simulink model "LQG_r"  (R2023b)
settings: Solver=VariableStepAuto  StartTime=0.0  StopTime=200  RelTol=1e-3
undefined symbols (not defined in the file): A, A_kf, B_kf, B_total, C_kf, C_ss, CI, D_kf, DI, DiscIntNeverNeededParam, Discrete, dVdt, K, Kint, Rn_ext, sigma, step_temp, steptime, Time, Ts, Tsp, Ufeedforward, Vb0, Vmax, Vmin, wd
libraries: simulink x3, ctrlSharedLib x1
settings Model: Creator=Maialen  LastModifiedBy=Maialen

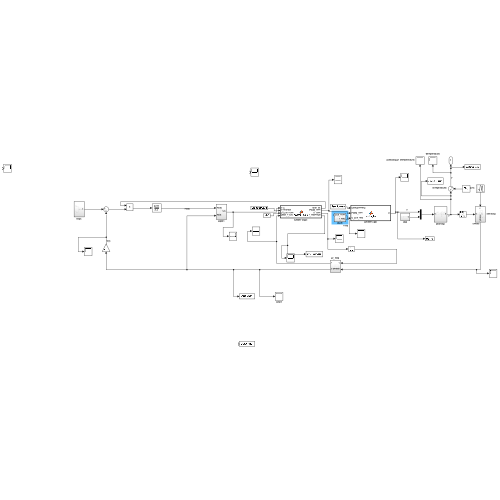
[thumbnail: Simulink's stored preview of the top-level diagram]
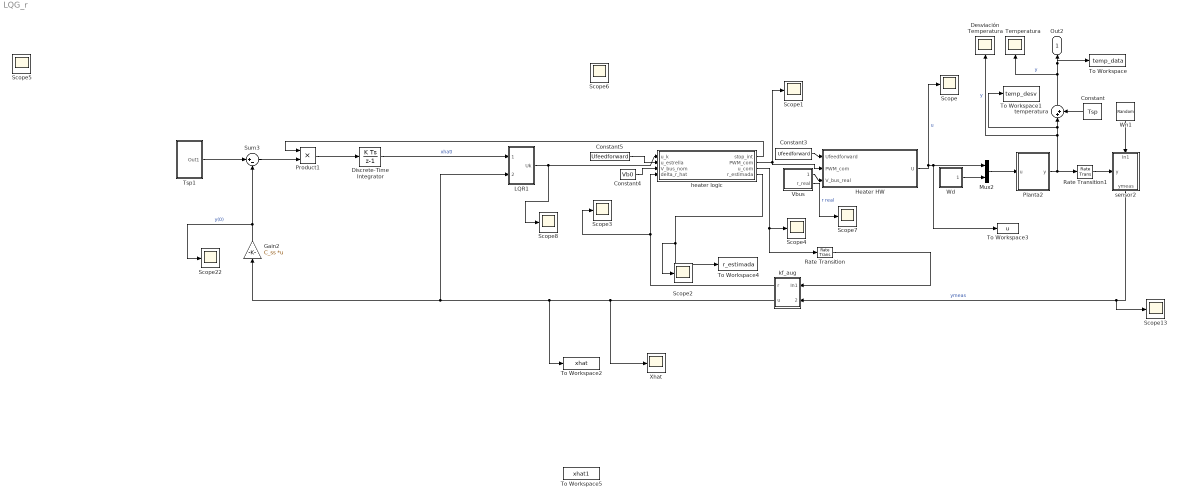
== system LQG_r ==
  Constant : Constant  Value=Tsp  SampleTime=0
  Constant3 : Constant  Value=Ufeedforward  SampleTime=0
  Constant4 : Constant  Value=Vb0  SampleTime=0
  Constant5 : Constant  Value=Ufeedforward  SampleTime=0
  Desviación Temperatura : Scope
  Discrete-Time Integrator : DiscreteIntegrator  SampleTime=Ts  ICPrevOutput=DiscIntNeverNeededParam  ICPrevScaledInput=DiscIntNeverNeededParam
  Gain2 : Gain  Gain=C_ss  Multiplication=Matrix(K*u)
  Heater HW : MATLAB Function  TreatAsAtomicUnit=on
  LQR1 : Subsystem
  Mux2 : Mux  Inputs=2
  Planta2 : Subsystem
  Product1 : Product
  Rate Transition : RateTransition  OutPortSampleTime=Ts
  Rate Transition1 : RateTransition  OutPortSampleTime=Ts
  Scope{,1..8,13,22} (11 alike) : Scope
  Sum3 : Sum  Inputs=|+-
  Temperatura : Scope
  To Workspace : ToWorkspace  VariableName=temp_data  SaveFormat=Timeseries  SampleTime=-1
  To Workspace1 : ToWorkspace  VariableName=temp_desv  SaveFormat=Timeseries  SampleTime=-1
  To Workspace2 : ToWorkspace  VariableName=xhat  SaveFormat=Timeseries  SampleTime=-1
  To Workspace3 : ToWorkspace  VariableName=u  SaveFormat=Timeseries  SampleTime=Ts
  To Workspace4 : ToWorkspace  VariableName=r_estimada  SaveFormat=Timeseries  SampleTime=-1
  To Workspace5 : ToWorkspace  VariableName=xhat1  SaveFormat=Timeseries  SampleTime=-1
  Tsp1 : Subsystem
  Vbus : Subsystem
  Wd : Subsystem
  Wn1 : RandomNumber  Variance=sigma^2  SampleTime=Ts
  Xhat : Scope
  heater logic : MATLAB Function  TreatAsAtomicUnit=on
  kf_aug : Subsystem
  sensor2 : Subsystem
      settings: PortSchema="{\"entries\":[{\"content\":{\"sides\":[{\"content\":{\"connectorIds\":[\"In1\"]},\"type\":\"ConnectorPlacement.EquallySpacedRectSide\",\"uuid\":\"87c57665-5a3a-4a29-be31-fc3b8356ea98\"},{\"content\":{\"connectorIds\":[\"Out1\"],\"side\":\"RIGHT\"},\"type\":\"ConnectorPlacement.EquallySpacedRectSide\",\"uuid\":\"3fe956b0-7f9e-4b46-bcb6-e49be4c7e683\"},{\"content\":{\"connectorIds\":[\"In2\"],\"side\":\"TOP\"},\"type\":\"ConnectorPlacement.EquallySpacedRectSide\",\"uuid\":\"3d207620-bc84-4c0d-9751-3dea453ac424\"}]},\"type\":\"ConnectorPlacement.EquallySpacedConnector\",\"uuid\":\"7e1a59fd-e04d-40d6-8549-9ebaaabea5d7\"}],\"packageUris\":[\"http://schema.mathworks.com/mf0/Connector/R2020b\"],\"version\":\"1.0\"}"
  temperatura : Sum  Inputs=|++
  Out2 : Outport
  wires:
  Vbus/2(r_real) -> Scope7/1  "r real"
  temperatura/1 -> To Workspace/1, Out2/1, Temperatura/1  "y"
  heater logic/3(u_com) -> Scope4/1, Rate Transition/1
  Vbus/1(V_bus_nom) -> Heater HW/3(V_bus_real)
  Heater HW/1(U) -> To Workspace3/1, Mux2/1, Scope/1  "u"
  Rate Transition1/1 -> sensor2/2(y)
  heater logic/4(r_estimada) -> To Workspace4/1, Scope2/1
  Rate Transition/1 -> kf_aug/1(In1)
  Constant3/1 -> Heater HW/1(Ufeedforward)
  Wd/1(Out1) -> Mux2/2
  Mux2/1 -> Planta2/1(u)
  Constant4/1 -> heater logic/3(V_bus_nom)
  Constant/1 -> temperatura/2
  Planta2/1(y) -> Desviación Temperatura/1, To Workspace1/1, temperatura/1, Rate Transition1/1  "y"
  kf_aug/2(u) -> To Workspace2/1, LQR1/2(xhat), Gain2/1, Xhat/1
  heater logic/2(PWM_com) -> Scope1/1, Heater HW/2(PWM_com)
  Constant5/1 -> heater logic/2(u_estrella)
  kf_aug/1(r) -> Scope3/1, heater logic/4(delta_r_hat)
  Wn1/1 -> sensor2/1(In1)
  sensor2/1(ymeas) -> kf_aug/2(ymeas), Scope13/1  "ymeas"
  LQR1/1(Uk) -> Scope8/1, heater logic/1(u_k)
  Discrete-Time Integrator/1 -> LQR1/1(xhatI)  "xhatI"
  Tsp1/1(Out1) -> Sum3/1
  Product1/1 -> Discrete-Time Integrator/1
  Sum3/1 -> Product1/2
  Gain2/1 -> Sum3/2, Scope22/1  "y(0)"
  heater logic/1(stop_int) -> Product1/1

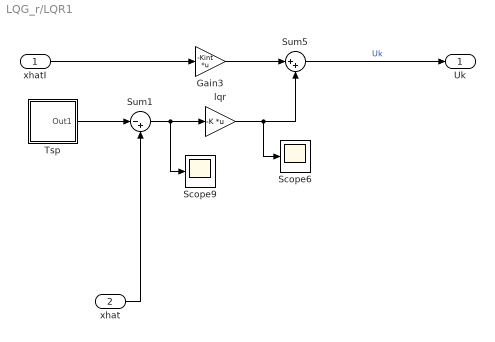
== system LQG_r/LQR1 ==
  xhatI : Inport
  xhat : Inport  Port=2
  Gain3 : Gain  Gain=-Kint  Multiplication=Matrix(K*u)
  Scope6 : Scope
  Scope9 : Scope
  Sum1 : Sum  Inputs=|-+
  Sum5 : Sum  Inputs=|++
  Tsp : Subsystem
  lqr : Gain  Gain=-K  Multiplication=Matrix(K*u)
  Uk : Outport
  wires:
  xhatI/1 -> Gain3/1
  lqr/1 -> Scope6/1, Sum5/2
  Gain3/1 -> Sum5/1
  Sum1/1 -> Scope9/1, lqr/1
  xhat/1 -> Sum1/2
  Tsp/1(Out1) -> Sum1/1
  Sum5/1 -> Uk/1  "Uk"

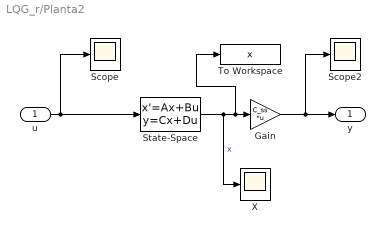
== system LQG_r/Planta2 ==
  u : Inport
  Gain : Gain  Gain=C_ss  Multiplication=Matrix(K*u)
  Scope : Scope
  Scope2 : Scope
  State-Space : StateSpace  A=A  B=B_total  C=CI  D=DI  InitialCondition=0
  To Workspace : ToWorkspace  VariableName=x  SaveFormat=Timeseries  SampleTime=-1
  X : Scope
  y : Outport
  wires:
  Gain/1 -> Scope2/1, y/1
  State-Space/1 -> X/1, To Workspace/1, Gain/1  "x"
  u/1 -> State-Space/1, Scope/1

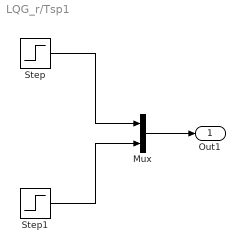
== system LQG_r/Tsp1 ==
  Mux : Mux  Inputs=2
  Step : Step  Time=steptime  After=step_temp  SampleTime=0
  Step1 : Step  Time=steptime  After=step_temp  SampleTime=0
  Out1 : Outport
  wires:
  Mux/1 -> Out1/1
  Step/1 -> Mux/1
  Step1/1 -> Mux/2

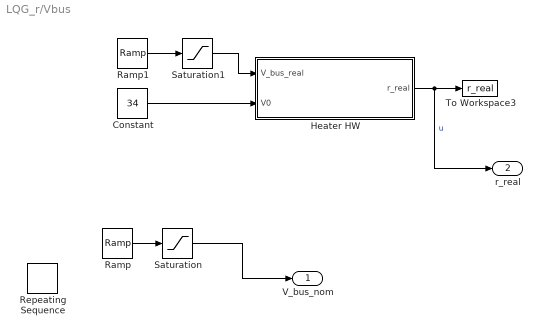
== system LQG_r/Vbus ==
  Constant : Constant  Value=34  SampleTime=0
  Heater HW : MATLAB Function  TreatAsAtomicUnit=on
  Ramp : simulink/Sources/Ramp  slope=dVdt  start=steptime  InitialOutput=Vb0
  Ramp1 : simulink/Sources/Ramp  slope=dVdt  start=steptime  InitialOutput=34
  Repeating Sequence : simulink/Sources/Repeating Sequence  rep_seq_t=[0, 20, 110, 310, 400, 600, 690, 890, 980]  rep_seq_y=[34, 34, 28, 28, 34, 34, 28, 28, 34]
  Saturation : Saturate  UpperLimit=Vmax  LowerLimit=Vmin
  Saturation1 : Saturate  UpperLimit=Vmax  LowerLimit=Vmin
  To Workspace3 : ToWorkspace  VariableName=r_real  SaveFormat=Timeseries  SampleTime=-1
  V_bus_nom : Outport
  r_real : Outport  Port=2
  wires:
  Constant/1 -> Heater HW/2(V0)
  Heater HW/1(r_real) -> r_real/1, To Workspace3/1  "u"
  Ramp/1 -> Saturation/1
  Saturation1/1 -> Heater HW/1(V_bus_real)
  Ramp1/1 -> Saturation1/1
  Saturation/1 -> V_bus_nom/1

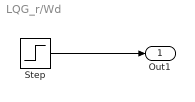
== system LQG_r/Wd ==
  Step : Step  Time=steptime  After=wd  SampleTime=0
  Out1 : Outport
  wires:
  Step/1 -> Out1/1

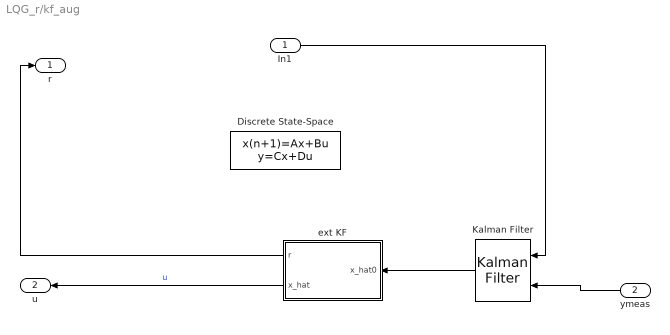
== system LQG_r/kf_aug ==
  In1 : Inport
  ymeas : Inport  Port=2
  Discrete State-Space : DiscreteStateSpace  A=A_kf  B=B_kf  C=C_kf  D=D_kf  SampleTime=Ts
  Kalman Filter : ctrlSharedLib/Kalman Filter  TimeDomain=Discrete-Time  UseCurrentEstimator=on  ModelSource=LTI State-Space Variable  ModelSourceVariable=syskf_ext  A=0.95  B=1  C=1  D=0  NumberOfStates=1  NumberOfInputs=1  NumberOfOutputs=1  InitialEstimateSource=Dialog  X0=0  P0=10  UseK=off  UseGH=off  NumberOfProcessNoiseInputs=1  G=1  TimeInvariantG=on  H=0  TimeInvariantH=on  Q=Qn_ext  TimeInvariantQ=on  R=Rn_ext  TimeInvariantR=on  N=0  TimeInvariantN=on  AddInputPort=on  AddEnablePort=off  OutputEstimatedY=off  OutputP=off  Ts=-1
  ext KF : MATLAB Function  TreatAsAtomicUnit=on
  r : Outport
  u : Outport  Port=2
  wires:
  ext KF/2(x_hat) -> u/1  "u"
  ext KF/1(r) -> r/1
  ymeas/1 -> Kalman Filter/2
  In1/1 -> Kalman Filter/1
  Kalman Filter/1 -> ext KF/1(x_hat0)

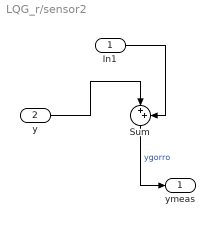
== system LQG_r/sensor2 ==
  In1 : Inport
  y : Inport  Port=2
  Sum : Sum  Inputs=|++
  ymeas : Outport
  wires:
  In1/1 -> Sum/2
  y/1 -> Sum/1
  Sum/1 -> ymeas/1  "ygorro"

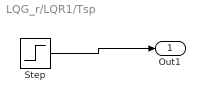
== system LQG_r/LQR1/Tsp ==
  Step : Step  Time=steptime  After=step_temp  SampleTime=0
  Out1 : Outport
  wires:
  Step/1 -> Out1/1

== matlab function LQG_r/Heater HW ==
  data: Ufeedforward input; PWM_com input; U output; V_bus_real input
function U = heater_hw(Ufeedforward, PWM_com, V_bus_real)
    R_real = [156.8; 156.8];
    
    % Potencia real entregada a la planta
    P_max_real = (V_bus_real^2) ./ R_real;
    U= PWM_com .* P_max_real - Ufeedforward;
end

== matlab function LQG_r/kf_aug/ext KF ==
  data: r output; x_hat0 input; x_hat output
function [r, x_hat] = ext(x_hat0)
   % x_hat es la salida del filtro (39x1)
x_hat = x_hat0(1:38); 
r = (x_hat0(39) ) ;

end

== matlab function LQG_r/Vbus/Heater HW ==
  data: V_bus_real input; V0 input; r_real output
function r_real = eficiencia_real(V_bus_real, V0)
    R_real = [156.8; 156.8];
    r_real = (V_bus_real/V0)^2;
end

== matlab function LQG_r/heater logic ==
  data: stop_int output; u_k input; u_estrella input; PWM_com output; V_bus_nom input; delta_r_hat input; u_com output; r_estimada output
function [stop_int, PWM_com, u_com, r_estimada] = heater_logic(u_k, u_estrella, V_bus_nom, delta_r_hat)
% u_k        : salida del controlador LQR (desviación de control)
% u_estrella : feedforward nominal (Ufeedforward)
% V_bus_nom  : voltaje nominal del bus (34V)
% delta_r_hat: estimación de Δr = r-1 del Kalman aumentado

    R0 = [156.8; 156.8];
    P_max_nom = (V_bus_nom^2) ./ R0;   % potencia máxima en nominal

   

    % Compensación feedforward de voltaje:
    % La caída de bus reduce la potencia disponible en u_estrella*Δr
    % El controlador compensa sumando esa pérdida estimada
    u_ff = -u_estrella .* delta_r_hat;   % (2×1) — negativo porque Δr<0 al caer

    % Potencia demandada total (control + feedforward nominal + compensación bus)
    P_demanda = u_estrella + u_k + u_ff;

    % Anti-windup: congela integrador si satura
    sat_arriba = P_demanda >= P_max_nom;
    sat_abajo  = P_demanda <= 0;
    stop_int   = double(~(sat_arriba | sat_abajo));

    % Saturación física
    P_limitada = max(0, min(P_max_nom, P_demanda));

    % PWM en voltaje nominal (heater_hw aplica el voltaje real)
    PWM_com = min(1, P_limitada ./ P_max_nom);

    % u_com: lo que realmente entra a la planta en desviaciones
    % (para logging, no vuelve al Kalman)
    u_com = P_limitada - u_estrella ;
    u_com = u_k +u_ff;
  

    r_estimada = delta_r_hat + 1;
end
